simulink subsystem "PieroControlado"  (R2023b)
settings: Solver=VariableStepAuto  StartTime=0.0  StopTime=10.0  RelTol=1e-3
settings Model: Creator=manu_  LastModifiedBy=manu_

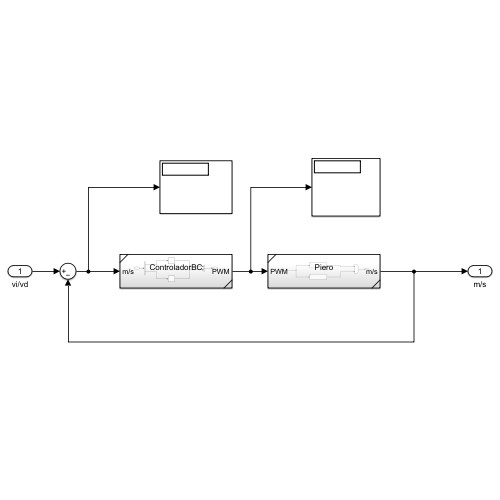
[thumbnail: Simulink's stored preview of the top-level diagram]
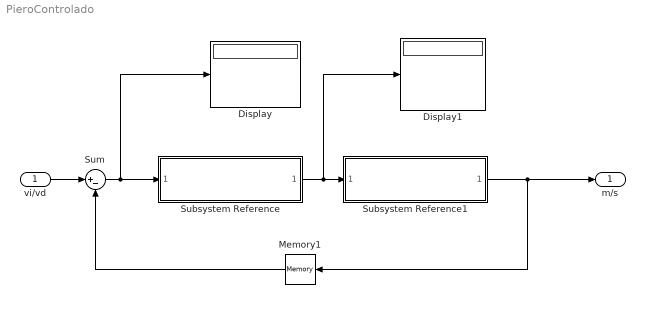
== system PieroControlado ==
  vi/vd : Inport
  Display : Display
  Display1 : Display
  Memory1 : Memory
  Subsystem Reference : Subsystem  ReferencedSubsystem=ControladorBC
  Subsystem Reference1 : Subsystem  ReferencedSubsystem=Piero
  Sum : Sum  Inputs=|+-
  m/s : Outport
  wires:
  vi/vd/1 -> Sum/1
  Sum/1 -> Display/1, Subsystem Reference/1
  Subsystem Reference/1 -> Display1/1, Subsystem Reference1/1
  Subsystem Reference1/1 -> Memory1/1, m/s/1
  Memory1/1 -> Sum/2
